simulink model "Autocorrelation"  (Simulink 7.8)
settings: Solver=ode45  StartTime=0.0  StopTime=10.0  RelTol=1e-3
values from neighbouring files (symbols this model uses):
  i = 3    [auto_correlation_data.mat]
  Ri = [0.12 0.01 0.23 0.28 0.89 0.31 0.64 0.28 0.83 0.93 0.33 0.15 ... (30 elements, 1x30)]    [auto_correlation_data.mat]
  Ztab = 1.96    [auto_correlation_data.mat]
libraries: simulink x1
settings Model: Creator=Windows  LastModifiedBy=Windows

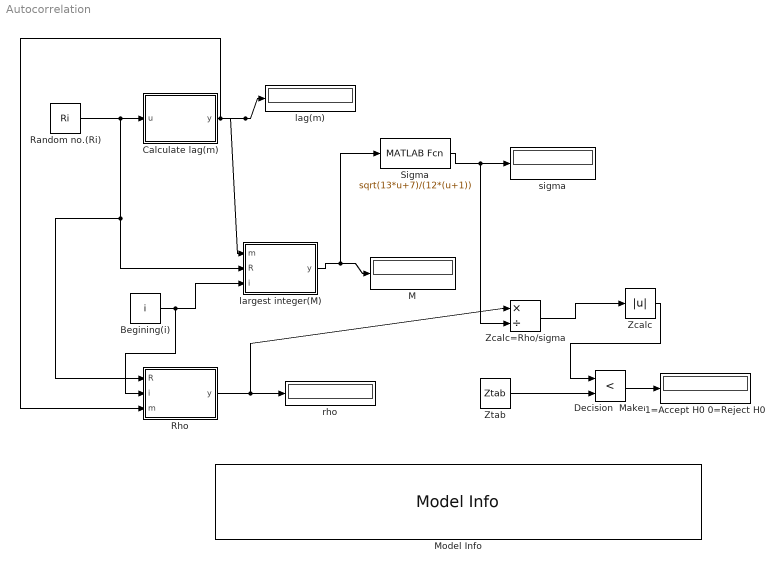
== system Autocorrelation ==
  1=Accept H0 0=Reject H0 : Display
  Begining(i) : Constant  Value=i
  Calculate lag(m) : MATLAB Function  TreatAsAtomicUnit=on
  Decision  Maker : RelationalOperator  Operator=<  OutDataTypeStr=boolean
  M : Display
  Model Info : simulink/Model-Wide Utilities/Model Info  InitialBlockCM=None  BlockCM=None  Frame=on  DisplayStringWithTags=|  HorizontalTextAlignment=Center  LeftAlignmentValue=0.5  SourceBlockDiagram=Autocorrelation  TagMaxNumber=20
      | Model Info
      | %<ModelName>
      | %<Created>
      | AutoCorrelation test helps to find out whether the random number to be tested are correlated or not.
      | The test statistic is based on normal distribution.
  Random no.(Ri) : Constant  Value=Ri
  Rho : MATLAB Function  TreatAsAtomicUnit=on
  Sigma : MATLABFcn  MATLABFcn=sqrt(13*u+7)/(12*(u+1))
  Zcalc : Abs
  Zcalc=Rho/sigma : Product  Inputs=*/
  Ztab : Constant  Value=Ztab
  lag(m) : Display
  largest integer(M) : MATLAB Function  TreatAsAtomicUnit=on
  rho : Display
  sigma : Display
  wires:
  Random no.(Ri)/1 -> Calculate lag(m)/1(u), largest integer(M)/2(R), Rho/1(R)
  Calculate lag(m)/1(y) -> lag(m)/1, largest integer(M)/1(m), Rho/3(m)
  Begining(i)/1 -> largest integer(M)/3(i), Rho/2(i)
  largest integer(M)/1(y) -> M/1, Sigma/1
  Sigma/1 -> sigma/1, Zcalc=Rho/sigma/2
  Rho/1(y) -> rho/1, Zcalc=Rho/sigma/1
  Zcalc=Rho/sigma/1 -> Zcalc/1
  Zcalc/1 -> Decision  Maker/1
  Ztab/1 -> Decision  Maker/2
  Decision  Maker/1 -> 1=Accept H0 0=Reject H0/1

== matlab function largest integer(M) ==
  data: m input double; y output double; R input double; i input double
function y = LargestM(m,R,i)
%#codegen
y=floor(((length(R)-i)/m)-1);

== matlab function Calculate lag(m) ==
  data: u input double; y output double
function y = lag(u)
%#codegen

z = zeros(1,1);
m = zeros(1,1);
for x=1:1:length(u)/6
    z=max(u(x));
    m=x;
end
y=m;

== matlab function Rho ==
  data: R input double; y output double; i input double; m input double
function y = Rho(R,i,m)
%#codegen
rho=zeros(1,1);
for k=1:1:5
    rho=rho+(1/5)*(R(i+(k-1)*m)*R(i+(k)*m));
end
rho=rho-0.25;
y = rho;
